simulink model "Test_PIL_IIR_Filter"  (R2017b)
settings: Solver=FixedStepDiscrete  StartTime=0.0  StopTime=1  FixedStep=0.001  RelTol=1e-3  EnableMultiTasking=on
PreLoadFcn:
  | run iir_startup;
model workspace (MAT data in the model file):
  dataint = Simulink.Signal
  dataint.DataType = 'int32'
  dataint.Dimensions = -1
  dataint.DimensionsMode = 'auto'
  dataint.Complexity = 'real'
  dataint.SampleTime = -1
  dataint.SamplingMode = 'auto'
  dataint.InitialValue = '0'
libraries: simulink x1
settings Model: DataTypeOverrideAppliesTo=Floating-point  Creator=obas  LastModifiedBy=Link
settings DataIOCC: ExternalInput=[t, testdata]  FinalStateName=xFinal_PIL  LoadExternalInput=on  SaveFormat=Array  SignalLoggingSaveFormat=ModelDataLogs  SignalLogging=off  StateSaveName=xout_PIL  TimeSaveName=tout_PIL  OutputSaveName=yout_PIL  SignalLoggingName=logsOut_PIL
settings OptimizationCC: ExpressionDepthLimit=2147483647  ZeroExternalMemoryAtStartup=off  ZeroInternalMemoryAtStartup=off  LifeSpan=1
settings DebuggingCC: SaveWithParameterizedLinksMsg=none  UnderspecifiedInitializationDetection=Classic  MergeDetectMultiDrivingBlocksExec=none  CheckExecutionContextPreStartOutputMsg=on  CheckExecutionContextRuntimeOutputMsg=on  SignalResolutionControl=TryResolveAllWithWarning  SolverPrmCheckMsg=warning  MultiTaskDSMMsg=warning  MultiTaskCondExecSysMsg=none  ParameterPrecisionLossMsg=none  StateNameClashWarn=warning  StrictBusMsg=ErrorOnBusTreatedAsVector  SFUnexpectedBacktrackingDiag=warning  SFNoUnconditionalDefaultTransitionDiag=warning  SFExecutionAtInitializationDiag=none
settings HardwareCC: ProdBitPerPointer=32  ProdBitPerSizeT=32  ProdBitPerPtrDiffT=32  ProdLargestAtomicInteger=Integer  ProdWordSize=32  ProdHWDeviceType=STMicroelectronics->STM32 32-bit Cortex-M
settings ModelReferenceCC: PropagateSignalLabelsOutOfModel=off
settings SFSimCC: SimUserSources=stm32f4xx_rcc  MATLABDynamicMemAlloc=off
settings RTWCC: SystemTargetFile=stm32.tlc  TemplateMakefile=stm32.tmf  Description=stm32 (Embedded Target)  GenerateReport=on  IncludeHyperlinkInReport=on  CreateSILPILBlock=PIL  CodeExecutionProfiling=on  CodeProfilingInstrumentation=on  GenerateCodeReplacementReport=on
settings CodeAppCC: IgnoreCustomStorageClasses=off  MaxIdLength=64  CustomSymbolStrType=$N$R$M  SimulinkBlockComments=off  InternalIdentifier=Classic
settings STFCustomTargetCC: CodeReplacementLibrary=ARM CMSIS SIN COS  ParMdlRefBuildCompliant=on  IncludeMdlTerminateFcn=off  CombineOutputUpdateFcns=on  ERTCustomFileBanners=on  SupportNonFinite=off  SupportComplex=off  SupportContinuousTime=off  SupportNonInlinedSFcns=off  RemoveResetFunc=on  MATLABClassNameForMDSCustomization=Simulink.SoftwareTarget.ERTCustomization  GRTInterface=off  SystemTargetFile=stm32.tlc
settings ERTTargetCC: CodeReplacementLibrary=ARM CMSIS SIN COS  MultiwordLength=2048  CompOptLevelCompliant=off  ConcurrentExecutionCompliant=off  IncludeMdlTerminateFcn=off  SupportNonFinite=off  SupportComplex=off  ModelStepFunctionPrototypeControlCompliant=off  CPPClassGenCompliant=off  UseToolchainInfoCompliant=off  ERTSrcFileBannerTemplate=sourceFileTemplate.cgt  ERTHdrFileBannerTemplate=sourceFileTemplate.cgt  ERTDataSrcFileTemplate=sourceFileTemplate.cgt  ERTDataHdrFileTemplate=sourceFileTemplate.cgt  ERTCustomFileTemplate=customRoutineProcess.tlc  ConvertIfToSwitch=off  SuppressUnreachableDefaultCases=off
settings ConfigComp: CovMetricSettings=dw  CovHtmlReporting=on  CovSaveCumulativeToWorkspaceVar=on  CovSaveSingleToWorkspaceVar=on  CovExternalEMLEnable=off  CovSFcnEnable=off

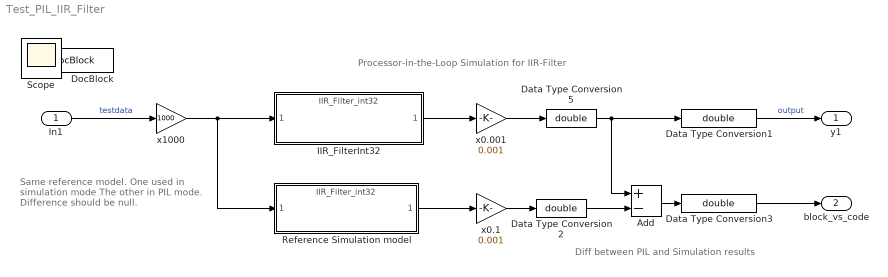
== system Test_PIL_IIR_Filter ==
  note: Same reference model.
      | One used in simulation mode
      | The other in PIL mode.
      | Difference should be null.
  note: Diff between PIL and Simulation results
  note: Processor-in-the-Loop Simulation for IIR-Filter
  In1 : Inport  OutDataTypeStr=double
  Add : Sum  Inputs=+-
  Data Type Conversion{1..3,5} (4 alike) : DataTypeConversion  OutDataTypeStr=double  SaturateOnIntegerOverflow=on  RndMeth=Zero
  DocBlock : simulink/Model-Wide Utilities/DocBlock  DocumentType=Text
      content=|
      | The model contains a 1st-order IIR filter of the following form:
      |
      |     y(n) = a1*y(n-1) + b0*u(n)
      |
      | Using the model pre-load function callback:
      |
      |     a1 = 0.9
      |     b0 = 0.1
      |
      | The filter is sampled at 1000Hz.
      |
      | Modified from iir_filter.mdl to enable ERT code generation.
  IIR_FilterInt32 : ModelReference  ModelNameDialog=IIR_Filter_int32.slx  SimulationMode=Processor-in-the-loop (PIL)  ModelReferenceVersion=1.107
  Reference Simulation model : ModelReference  ModelNameDialog=IIR_Filter_int32.slx  SimulationMode=Normal  ModelReferenceVersion=1.107
  x0.001 : Gain  Gain=0.001
  x0.1 : Gain  Gain=0.001
  x1000 : Gain  Gain=1000  ParamDataTypeStr=uint32  OutMin=-2147483647-1  OutMax=2147483647  OutDataTypeStr=int32
  y1 : Outport
  block_vs_code : Outport  Port=2
  Scope : Scope
  wires:
  In1/1 -> x1000/1  "testdata"
  Data Type Conversion1/1 -> y1/1  "output"
  Data Type Conversion3/1 -> block_vs_code/1
  Add/1 -> Data Type Conversion3/1
  Data Type Conversion5/1 -> Add/1, Data Type Conversion1/1
  x0.001/1 -> Data Type Conversion5/1
  x1000/1 -> Reference Simulation model/1, IIR_FilterInt32/1
  IIR_FilterInt32/1 -> x0.001/1
  x0.1/1 -> Data Type Conversion2/1
  Reference Simulation model/1 -> x0.1/1
  Data Type Conversion2/1 -> Add/2
